simulink model "tracking3"  (R2023b)
settings: Solver=VariableStepAuto  StartTime=0.0  StopTime=20  FixedStep=0.01  RelTol=1e-3
libraries: spsSeriesRLCBranchLib x6, spsDiodeLib x2, spsVoltageMeasurementLib x2, simulink x2, spsControlledVoltageSourceLib x1, spsCurrentMeasurementLib x1, spsMosfetLib x1, slpidlib x1, spsPWMGeneratorDCDCLib x1, spsPVArrayLib x1, sps_lib x1
settings Model: Creator=Dong  LastModifiedBy=yeowy
settings SolverCC: AlgebraicLoopSolver=TrustRegion
settings DebuggingCC: UnconnectedInputMsg=warning  UnconnectedOutputMsg=warning  UnconnectedLineMsg=warning
settings ModelReferenceCC: EnableRefExpFcnMdlSchedulingChecks=on
settings SFSimCC: CustomCodeUndefinedFunction=UseInterfaceOnly

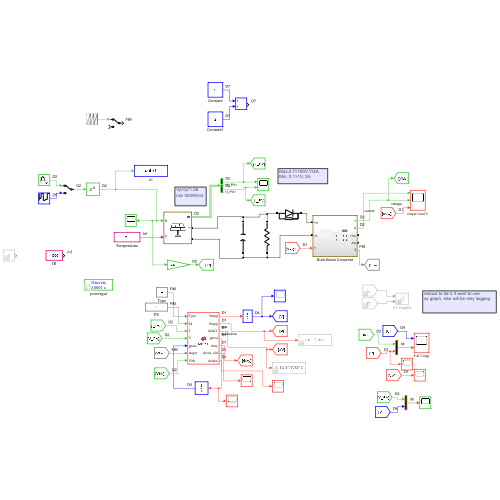
[thumbnail: Simulink's stored preview of the top-level diagram]
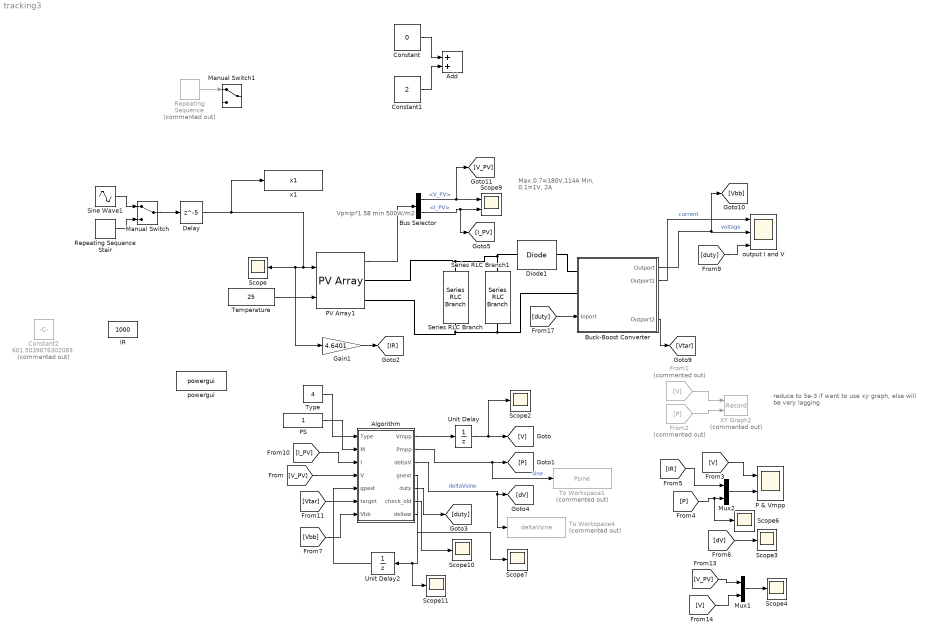
== system tracking3 ==
  note: Vp=Ip*1.58
      | min 500W/m2
  note: Max,0.7=180V,114A
      | Min, 0.1=1V, 2A
  note: reduce to 5e-3 if want to use
      | xy graph, else will be very lagging
  Add : Sum
  Algorithm : MATLAB Function  TreatAsAtomicUnit=on
  Buck-Boost Converter : Subsystem
      settings: PortSchema="{\"entries\":[{\"content\":{\"sides\":[{\"content\":{\"connectorIds\":[\"LConn1\",\"LConn2\",\"In1\"]},\"type\":\"ConnectorPlacement.EquallySpacedRectSide\",\"uuid\":\"434e697c-d5be-45e6-bdc1-8ae755998e80\"},{\"content\":{\"connectorIds\":[\"Out1\",\"Out2\",\"RConn1\",\"RConn2\",\"Out3\"],\"side\":\"RIGHT\"},\"type\":\"ConnectorPlacement.EquallySpacedRectSide\",\"uuid\":\"10395034-5ec3-4cb8-9f4e-a5ff74166f8a\"},{\"content\":{\"side\":\"TOP\"},\"type\":\"ConnectorPlacement.EquallySpacedRectSide\",\"uuid\":\"7465b0d6-f669-4ab3-bc57-21c5b1d9d369\"}]},\"type\":\"ConnectorPlacement.EquallySpacedConnector\",\"uuid\":\"ddac4feb-4ed3-480d-95df-f0f80e961ae6\"}],\"packageUris\":[\"http://schema.mathworks.com/mf0/Connector/R2020b\"],\"version\":\"1.0\"}"
  Bus Selector : BusSelector  OutputSignals=V_PV,I_PV
  Constant : Constant  Value=0  VectorParams1D=off  SampleTime=1
  Constant1 : Constant  Value=2  VectorParams1D=off  SampleTime=1
  Constant2 : Constant  Commented=on  Value=601.5039876302083
  Delay : Delay  DelayLength=5
  Diode1 : spsDiodeLib/Diode  Ron=0.001  Lon=0  Vf=10  IC=0  UseSnubber=0  Rs=500  Cs=250e-9  Measurements=off
  From1 : From  Commented=on  GotoTag=V
  From2 : From  Commented=on  GotoTag=P
  Gain1 : Gain  Gain=4.6401
  IR : Constant  Value=1000
  Manual Switch : ManualSwitch
  Manual Switch1 : ManualSwitch
  Mux1 : Mux  Inputs=2
  Mux2 : Mux  Inputs=2
  P & Vmpp : Scope  NumInputPorts=2
  PS : Constant  SampleTime=0
  PV Array1 : spsPVArrayLib/PV Array  Npar=4  Nser=2  PlotType=array @ 25 deg.C & specified irradiances  S_vec="[ 1000  500  100 ]"  Temp_C_vec="[ 45 25  ]"  ModuleName=User-defined  PlotWhenSelected=off  Pm=580.0124  Ncell=144  Voc=51.4  Isc=14.22  Vm=43.22  Im=13.42  beta_Voc_pc=-0.36099  alpha_Isc_pc=0.102  beta_Voc=-0.18555  alpha_Isc=0.014504  IL=14.2363  I0=5.2538e-10  nI=0.5786  Rsh=331.4965  Rs=0.12745  RobustModel=off  RobustCellTemperature=313.3991  BAL=on  Tc=1e-6  Tfilter=5e-5
  Repeating Sequence : simulink/Sources/Repeating Sequence  Commented=on  rep_seq_t=[0 0.1]  rep_seq_y=[2 10]*100
  Repeating Sequence Stair : simulink/Sources/Repeating Sequence Stair  OutValues=[6 10 4 5 10].'*100  tsamp=0.05  OutMin=[]  OutMax=[]  OutDataTypeStr=double  OutputDataTypeScalingMode=double  OutDataType=fixdt(0,8)  ConRadixGroup=Best Precision: Vector-wise  OutScaling=2^-12
  Scope{,2..4,6..7,10..11} (8 alike) : Scope
  Scope9 : Scope  NumInputPorts=2
  Series RLC Branch : spsSeriesRLCBranchLib/Series RLC Branch  LConnTagsString=__new0  RConnTagsString=__new0  BranchType=C  Resistance=2  Inductance=1e-3  SetiL0=off  InitialCurrent=0  Capacitance=1e-3  Setx0=off  InitialVoltage=0  Measurements=None
  Series RLC Branch1 : spsSeriesRLCBranchLib/Series RLC Branch  LConnTagsString=__new0  RConnTagsString=__new0  BranchType=R  Resistance=80  Inductance=1e-3  SetiL0=off  InitialCurrent=0  Capacitance=1e-5  Setx0=off  InitialVoltage=0  Measurements=None
  Sine Wave1 : Sin  Amplitude=200  Bias=800  Frequency=3.14*3  Samples=2  SampleTime=1e-4
  Temperature : Constant  Value=25
  To Workspace1 : ToWorkspace  Commented=on  VariableName=Psine  SaveFormat=Timeseries  SampleTime=-1
  To Workspace4 : ToWorkspace  Commented=on  VariableName=deltaVsine  SaveFormat=Timeseries  SampleTime=-1
  Type : Constant  Value=4  SampleTime=0
  Unit Delay : UnitDelay  InitialCondition=0.1  SampleTime=0.001  HasFrameUpgradeWarning=on
  Unit Delay2 : UnitDelay  InitialCondition=0.1  SampleTime=0.001  HasFrameUpgradeWarning=on
  XY Graph2 : Record  Commented=on  FileSettingsInternal="{\"entries\":[{\"content\":{\"excelSettings\":{\"content\":{},\"type\":\"Streamout.ExcelSettings\"}},\"type\":\"Streamout.FileSettingStorage\",\"uuid\":\"\"}],\"packageUris\":[\"http:\\/\\/schema.mathworks.com\\/mf0\\/streamout_blocks\\/R2020a\"],\"version\":\"1.0\"}"  Layout=[1 1]  SignalsInternal="{\"entries\":[{\"content\":{},\"type\":\"RecordBlkView.InputSignals\",\"uuid\":\"\"}],\"packageUris\":[\"http:\\/\\/schema.mathworks.com\\/mf0\\/streamout_blocks\\/R2020a\"],\"version\":\"1.0\"}"  VisualizationBindings="{\"xyplotplugin\":{\"info\":[{\"series\":[],\"subplotID\":1}]}}"  CompatibilityTag=XY
  output I and V : Scope  NumInputPorts=3
  powergui : sps_lib/powergui  Priority=1  SimulationMode=Discrete  SampleTime=1e-4  frequency=60  Iterations=50  frequencyindice=0  Pbase=100e6  ErrMax=1e-4  UnitsV=kV  UnitsW=MW  buscounter=0  FunctionMessages=off  echomessages=off  EnableUseOfTLC=off  CurrentSourceSwitches=off  DisableSnubberDevices=off  DisableRonSwitches=off  DisableVfSwitches=off  DisplayEquations=off  AutomaticDiscreteSolvers=off  SolverType=Backward Euler  Interpol=off  ExternalGateDelay=off  methode=off  Ts=0  x0status=blocks  SPID=off  SwTol=0  HookPort=off  NonlinearTolerance=1e-4  nMaxIteration=100  ContinueOnMaxIteration=off  RestoreLinks=warning  ResistiveCurrentMeasurement=off  Frange=[0:2:500]  Ylog=off  Xlog=on  ShowGrid=off  save=off  variable=ZData  structure=0  ZoomFFT=off  StartTime=0.0  cycles=1  DisplayStyle=1  fundamental=60  FreqAxis=off  MaxFrequency=1000  frequencyindicesteady=1  RmsSteady=1  display=off
  x1 : ToWorkspace  VariableName=x1  SampleTime=1
      settings: Save2DSignal=2-D array (concatenate along first dimension)
  wires:
  Constant/1 -> Add/1
  Constant1/1 -> Add/2
  [Vtar] -> Algorithm/6(target)
  [V_PV] -> Algorithm/4(V)
  Repeating Sequence/1 -> Manual Switch1/1
  Repeating Sequence Stair/1 -> Manual Switch/2
  [V_PV] -> Mux1/1
  Sine Wave1/1 -> Manual Switch/1
  Manual Switch/1 -> Delay/1
  [I_PV] -> Algorithm/3(I)
  [duty] -> output I and V/3
  Buck-Boost Converter/3(Outport2) -> [Vtar]
  Algorithm/3(deltaV) -> To Workspace4/1, [dV]  "deltaVsine"
  [V] -> Mux1/2
  Mux1/1 -> Scope4/1
  [V] -> P & Vmpp/1
  Bus Selector/1 -> [V_PV], Scope9/1  "<V_PV>"
  [dV] -> Scope3/1
  Buck-Boost Converter/2(Outport1) -> output I and V/1  "current"
  Bus Selector/2 -> [I_PV], Scope9/2  "<I_PV>"
  Mux2/1 -> P & Vmpp/2
  From2/1 -> XY Graph2/2
  Algorithm/5(duty) -> [duty]
  [IR] -> Mux2/1
  [P] -> Scope6/1, Mux2/2
  [Vbb] -> Algorithm/7(Vbb)
  Algorithm/6(check_old) -> Scope10/1
  Algorithm/2(Pmpp) -> To Workspace1/1, [P]  "sine"
  Algorithm/7(deltaw) -> Scope7/1
  PS/1 -> Algorithm/2(M)
  Unit Delay/1 -> Scope2/1, [V]
  [duty] -> Buck-Boost Converter/1(Inport)
  PV Array1/1 -> Bus Selector/1
  Unit Delay2/1 -> Algorithm/5(gpast)
  Type/1 -> Algorithm/1(Type)
  Buck-Boost Converter/1(Outport) -> [Vbb], output I and V/2  "voltage"
  Algorithm/4(gnext) -> Scope11/1, Unit Delay2/1
  From1/1 -> XY Graph2/1
  Algorithm/1(Vmpp) -> Unit Delay/1
  Gain1/1 -> [IR]
  Temperature/1 -> PV Array1/2
  Delay/1 -> PV Array1/1, Gain1/1, Scope/1, x1/1
  connections:
  Series RLC Branch/LConn1 -- PV Array1/RConn1 -- Series RLC Branch1/LConn1 -- Diode1/LConn1
  Buck-Boost Converter/LConn2 -- Series RLC Branch1/RConn1 -- PV Array1/RConn2 -- Series RLC Branch/RConn1
  Diode1/RConn1 -- Buck-Boost Converter/LConn1

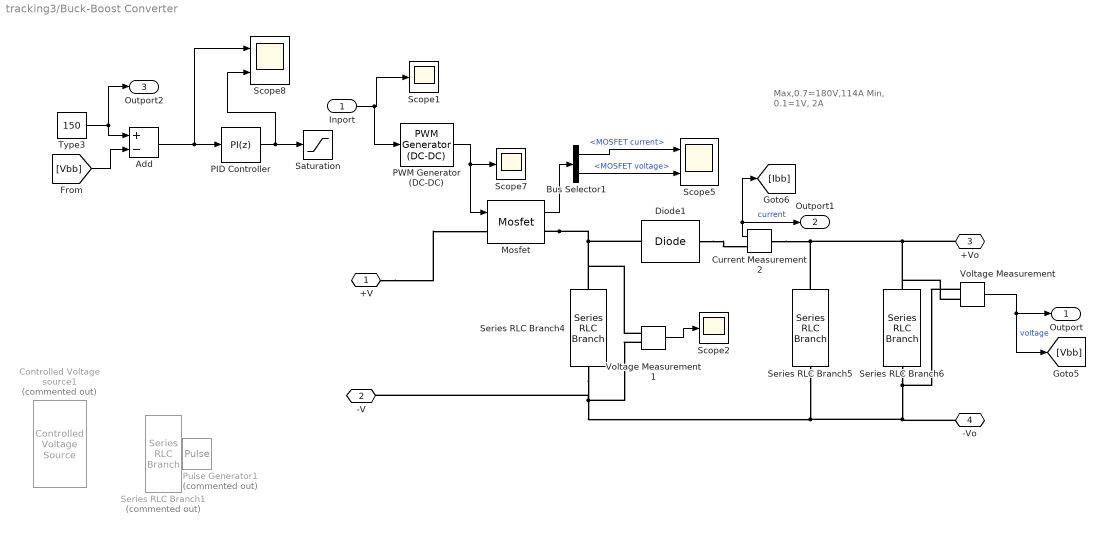
== system tracking3/Buck-Boost Converter ==
  note: Max,0.7=180V,114A
      | Min, 0.1=1V, 2A
  Inport : Inport
  Add : Sum  Inputs=+-
  Bus Selector1 : BusSelector  OutputSignals=MOSFET current,MOSFET voltage
  Controlled Voltage source1 : spsControlledVoltageSourceLib/Controlled Voltage Source  Commented=on  Initialize=on  Source_Type=DC  Amplitude=0  Phase=0  Frequency=0  Measurements=None
  Current Measurement2 : spsCurrentMeasurementLib/Current Measurement  PhasorSimulation=off  OutputType=Complex  PSBequivalent=0
  Diode1 : spsDiodeLib/Diode  Ron=0.001  Lon=0  Vf=0.8  IC=0  UseSnubber=0  Rs=500  Cs=250e-9  Measurements=off
  Mosfet : spsMosfetLib/Mosfet  Ron=0.1  Lon=0  Rd=0.01  Vfd=0  IC=0  Rs=1e5  Cs=inf  Measurements=on
  PID Controller : slpidlib/PID Controller  Controller=PI  Form=Parallel  TimeDomain=Discrete-time  UseExternalTs=off  SampleTime=-1  IntegratorMethod=Forward Euler  FilterMethod=Forward Euler  ControllerParametersSource=internal  P=0.448206848938492  I=8.01083955194228  UseKiTs=off  D=0  N=100  UseFilter=on  TunerSelectOption=Transfer Function Based (PID Tuner App)  InitialConditionSource=internal  InitialConditionForIntegrator=0  InitialConditionForFilter=0  DifferentiatorICPrevScaledInput=0  ExternalReset=none  TrackingMode=off  Kt=1  LimitOutput=on  SatLimitsSource=internal  UpperSaturationLimit=0.8  LowerSaturationLimit=0  LinearizeAsGain=off  AntiWindupMode=none  Kb=1  LimitIntegrator=on  UpperIntegratorSaturationLimit=0.8  LowerIntegratorSaturationLimit=0  POutMin=[]  POutMax=[]  IOutMin=[]  IOutMax=[]  DOutMin=[]  DOutMax=[]  NOutMin=[]  NOutMax=[]  SumOutMin=[]  SumOutMax=[]  SaturationOutMin=[]  SaturationOutMax=[]  PParamMin=[]  PParamMax=[]  IParamMin=[]  IParamMax=[]  DParamMin=[]  DParamMax=[]  NParamMin=[]  NParamMax=[]  KbParamMin=[]  KbParamMax=[]  KtParamMin=[]  KtParamMax=[]  KbOutMin=[]  KbOutMax=[]  KtOutMin=[]  KtOutMax=[]  IntegratorOutMin=[]  IntegratorOutMax=[]  FilterOutMin=[]  FilterOutMax=[]  SumI1OutMin=[]  SumI1OutMax=[]  SumI2OutMin=[]  SumI2OutMax=[]  SumI3OutMin=[]  SumI3OutMax=[]  SumI4OutMin=[]  SumI4OutMax=[]  SumDOutMin=[]  SumDOutMax=[]  DifferentiatorOutMin=[]  DifferentiatorOutMax=[]  FilterDiffOutCoefMin=[]  FilterDiffOutCoefMax=[]  ReciprocalOutMin=[]  ReciprocalOutMax=[]  SumDenOutMin=[]  SumDenOutMax=[]  SumNumOutMin=[]  SumNumOutMax=[]  DivideOutMin=[]  DivideOutMax=[]  UdiffTsProdOutMin=[]  UdiffTsProdOutMax=[]  NTsProdOutMin=[]  NTsProdOutMax=[]  UintegralTsProdOutMin=[]  UintegralTsProdOutMax=[]  UngainTsProdOutMin=[]  UngainTsProdOutMax=[]  ClampingZeroOutDataTypeStr=Inherit: Inherit via back propagation  ClampingZeroOutMin=[]  ClampingZeroOutMax=[]  FilterDenConstantOutDataTypeStr=Inherit: Inherit via back propagation  FilterDenConstantOutMin=[]  FilterDenConstantOutMax=[]  PCopyOutDataTypeStr=Inherit: Inherit via back propagation  PCopyOutMin=[]  PCopyOutMax=[]  NCopyOutDataTypeStr=Inherit: Inherit via back propagation  NCopyOutMin=[]  NCopyOutMax=[]  IntegratorContinuousStateAttributes=''  IntegratorStateMustResolveToSignalObject=off  IntegratorRTWStateStorageClass=Auto  FilterContinuousStateAttributes=''  FilterStateMustResolveToSignalObject=off  FilterRTWStateStorageClass=Auto  ParallelPVariant=InternalParameters  IdealPVariant=Disabled  IVariant=InternalParameters  DVariant=Disabled  IntegratorVariant=Discrete  SatVariant=Enabled  AWVariant=Passthrough  PCopyVariant=Disabled  TRVariant=Disabled  FdbkBlocksVariant=Forward  IdealPFdbkVariant=Disabled  SatFdbkVariant=Disabled  DerivativeFilterVariant=Disabled  NVariant=Disabled  NCopyVariant=Disabled_SignalSpec  FilterICVariant=Disabled  IntegratorICVariant=InternalICs  ExternalResetVariant=Disabled  TRSumVariant=Passthrough  SumFdbkVariant=Disabled  SumVariant=Sum_PI  TsampFilterVariant=InternalTs  TsampNgainVariant=Passthrough  TsampIntegralVariant=Disabled_SignalSpec  ExternalSaturationOutDataTypeStr=Inherit: Same as second input
  PWM Generator (DC-DC) : spsPWMGeneratorDCDCLib/PWM Generator (DC-DC)  Fsw=900  Ts=0
  Pulse Generator1 : DiscretePulseGenerator  Commented=on  Period=10  PulseWidth=8  SampleTime=5e-6
  Saturation : Saturate  UpperLimit=0.8  LowerLimit=0
  Scope1 : Scope
  Scope2 : Scope
  Scope5 : Scope  NumInputPorts=2
  Scope7 : Scope
  Scope8 : Scope  NumInputPorts=2
  Series RLC Branch1 : spsSeriesRLCBranchLib/Series RLC Branch  Commented=on  LConnTagsString=__new0  RConnTagsString=__new0  BranchType=L  Resistance=1  Inductance=8e-2  SetiL0=off  InitialCurrent=0  Capacitance=1e-6  Setx0=off  InitialVoltage=0  Measurements=None
  Series RLC Branch4 : spsSeriesRLCBranchLib/Series RLC Branch  LConnTagsString=__new0  RConnTagsString=__new0  BranchType=L  Resistance=1  Inductance=1e-3  SetiL0=off  InitialCurrent=0  Capacitance=1e-6  Setx0=off  InitialVoltage=0  Measurements=None
  Series RLC Branch5 : spsSeriesRLCBranchLib/Series RLC Branch  LConnTagsString=__new0  RConnTagsString=__new0  BranchType=C  Resistance=1  Inductance=1e-3  SetiL0=off  InitialCurrent=0  Capacitance=1e-2  Setx0=off  InitialVoltage=0  Measurements=None
  Series RLC Branch6 : spsSeriesRLCBranchLib/Series RLC Branch  LConnTagsString=__new0  RConnTagsString=__new0  BranchType=R  Resistance=50  Inductance=1e-3  SetiL0=off  InitialCurrent=0  Capacitance=1e-6  Setx0=off  InitialVoltage=0  Measurements=None
  Type3 : Constant  Value=150  SampleTime=0
  Voltage Measurement : spsVoltageMeasurementLib/Voltage Measurement  PhasorSimulation=off  OutputType=Complex  PSBequivalent=0
  Voltage Measurement1 : spsVoltageMeasurementLib/Voltage Measurement  PhasorSimulation=off  OutputType=Complex  PSBequivalent=0
  +V : PMIOPort  Side=Left
  -V : PMIOPort  Port=2  Side=Left
  +Vo : PMIOPort  Port=3  Side=Right
  -Vo : PMIOPort  Port=4  Side=Right
  Outport : Outport
  Outport1 : Outport  Port=2
  Outport2 : Outport  Port=3
  wires:
  [Vbb] -> Add/2
  Voltage Measurement/1 -> [Vbb], Outport/1  "voltage"
  Bus Selector1/1 -> Scope5/1  "<MOSFET current>"
  Voltage Measurement1/1 -> Scope2/1
  Bus Selector1/2 -> Scope5/2  "<MOSFET voltage>"
  PID Controller/1 -> Scope8/2, Saturation/1
  Add/1 -> Scope8/1, PID Controller/1
  Current Measurement2/1 -> [Ibb], Outport1/1  "current"
  Type3/1 -> Outport2/1, Add/1
  PWM Generator (DC-DC)/1 -> Mosfet/1, Scope7/1
  Mosfet/1 -> Bus Selector1/1
  Inport/1 -> PWM Generator (DC-DC)/1, Scope1/1
  connections:
  Series RLC Branch6/RConn1 -- -Vo/RConn1 -- Series RLC Branch4/RConn1 -- -V/RConn1 -- Voltage Measurement1/LConn2 -- Series RLC Branch5/LConn1 -- Voltage Measurement/LConn1
  Mosfet/RConn1 -- Diode1/RConn1 -- Voltage Measurement1/LConn1 -- Series RLC Branch4/LConn1
  Series RLC Branch5/RConn1 -- +Vo/RConn1 -- Voltage Measurement/LConn2 -- Series RLC Branch6/LConn1 -- Current Measurement2/LConn1
  Diode1/LConn1 -- Current Measurement2/RConn1
  +V/RConn1 -- Mosfet/LConn1

== matlab function tracking3/Algorithm ==
  settings: updateMethod=DISCRETE
  data: Type input; M input; I input; Vmpp output; V input; Pmpp output; deltaV output; gpast input; gnext output; duty output; target input; Vbb input; check_old output; deltaw output
function [Vmpp,Pmpp,deltaV, gnext, duty, check_old,deltaw] = MPPT(Type,M,I,V,gpast, target, Vbb)
%% MPPT TESTER FUNCTION
% Select one of the following Perturb & Observe algorithms, by setting Type
% Type=1 for FIXED STEP SIZE
% Type=2 for dP/dV STEP SIZE
% Type=3 for Auto-Scaling
% V input = PV array terminal voltage (V)
% I input = PV array current (A)
%%

duty_init = 0.1;
check=0;
% min and max value are used to limit duty between
% 0 and 0.85
delta=1e-4; %in steady state
duty_min=0;
duty_max=0.8;
deltaV=1;

persistent Vpast Ipast Ppast duty_old;
    if isempty(Vpast) % Setup some initial values
        Vpast=0.000001;
        Ipast=0.000001;
        
        %gpast=1;
        duty_old=duty_init;
        Ppast=Vpast*Ipast;
    end

deltaV=0; % initializing
P= V*I; % Measure Power for current iteration 
dI= I - Ipast;
dV= V - Vpast;
dP= P - Ppast;
g=abs(dP);
gpast=abs(gpast);
gup=gpast*1.1;
glow=gpast*0.8;

%% Define DeltaV for fixed perturbation-step MPPT [1]
    if (Type==1)  
        % suggested range of M;  0.3 @ 1000m/m2 and 0.7 @ 200m/m2
        delta = delta;
    %% Define DeltaV for variable perturbation-step MPPT [2]   
    elseif (Type==2)
        % suggested range of M; 0.3 @ 1000m/m2 and 0.7 @ 200m/m2
        deltaV = M*abs(dP/dV);
    %% Define DeltaV for auto-scaling technique MPPT [3]    
    elseif (Type==3)  
        % suggested value of M is 3 for all irridiance conditions
        F=1-(abs(I/V)/abs(dI/dV));
        G=1-(abs(dI/dV)/abs(I/V));
            if dP > 0
                if dV > 0
                    deltaV = M*G;
                else
                    deltaV = M*F;
                end
            else
                if dV > 0
                    deltaV = M*F;
                else
                    deltaV = M*G;
                end    
            end
    %%%%%%%%%%%%%%%%%%%%%%%%%%%%%%%%%%%%%%%%%%%%%%%%%%%%%%%%%%
    elseif (Type ==4)
        if (g>=glow && g<gup)
            delta=delta;   %used to track linear mpp
            check=0;
        elseif g>= gup
            %deltaV=3.41*abs(dI*V*(dV/dP));
            delta=(1e-4)*abs(dV*I*(dI/dP));  %used to track curve mpp          
            check=1;
        else
            delta=0;
        end
    elseif(Type==0)
        delta=0;       %ignore the selection
    end

%% MPPT Algorithm  
if dP ~= 0
    if dP < 0
        if dV < 0
            Vmpp = V + deltaV;
            if Vbb < target
                duty=duty_old + delta;
            elseif Vbb > target
                duty=duty_old - delta;
            else
                duty=duty_old;
            end
        else
            Vmpp = V - deltaV;
            if Vbb < target
                duty=duty_old + delta;
            elseif Vbb > target
                duty=duty_old - delta;
            else
                duty=duty_old;
            end
        end
    else
        if dV < 0
            Vmpp = V - deltaV;
            if Vbb < target
                duty=duty_old + delta;
            elseif Vbb > target
                duty=duty_old - delta;
            else
                duty=duty_old;
            end
        else
            Vmpp = V + deltaV;
            if Vbb < target
                duty=duty_old + delta;
            elseif Vbb > target
                duty=duty_old - delta;
            else
                duty=duty_old;
            end
        end    
    end
else
    Vmpp = V;
    duty=duty_old;
end

%%%next task use Vmpp to control duty

% if Vbb < target
%     duty=duty_old+delta;
% elseif Vbb > target
%     duty=duty_old-delta;
% else
%     duty=duty_old;
% end

%the below if limits the duty between min and max
if duty > duty_max
    duty=duty_max;
elseif duty<duty_min
    duty=duty_min;
end     

Pmpp=Vmpp*I;

%%
% Update Past values
duty_old=duty;
Vpast=V;
Ppast=P;
Ipast=I;
gnext = g;
check_old=check;
deltaw=delta;
end
